simulink model "Aufgabenliste_digital_2_simulink"  (R2015a)
settings: Solver=ode4  StartTime=0.0  StopTime=10.0  FixedStep=0.001  RelTol=1e-3
values from neighbouring files (symbols this model uses):
  A1 = 10    [Aufgabenliste_digital_2.m]
  A2 = 1    [Aufgabenliste_digital_2.m]
  w1 = 2*pi/10    (= 0.628318530718)    [Aufgabenliste_digital_2.m]
  w2 = 2*pi/0.1    (= 62.8318530718)    [Aufgabenliste_digital_2.m]
settings Model: Creator=daniel  LastModifiedBy=daniel

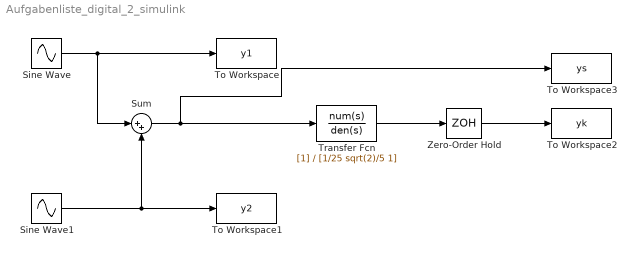
== system Aufgabenliste_digital_2_simulink ==
  Sine Wave : Sin  Amplitude=A1  Frequency=w1  SampleTime=0
  Sine Wave1 : Sin  Amplitude=A2  Frequency=w2  SampleTime=0
  Sum : Sum  Inputs=|++
  To Workspace : ToWorkspace  VariableName=y1  SaveFormat=Timeseries  SampleTime=-1
  To Workspace1 : ToWorkspace  VariableName=y2  SaveFormat=Structure With Time  SampleTime=-1
  To Workspace2 : ToWorkspace  VariableName=yk  SaveFormat=Structure With Time  SampleTime=-1
  To Workspace3 : ToWorkspace  VariableName=ys  SaveFormat=Structure With Time  SampleTime=-1
  Transfer Fcn : TransferFcn  Denominator=[1/25 sqrt(2)/5 1]
  Zero-Order Hold : ZeroOrderHold  SampleTime=0.11
  wires:
  Sine Wave/1 -> To Workspace/1, Sum/1
  Sine Wave1/1 -> To Workspace1/1, Sum/2
  Sum/1 -> Transfer Fcn/1, To Workspace3/1
  Zero-Order Hold/1 -> To Workspace2/1
  Transfer Fcn/1 -> Zero-Order Hold/1
